simulink model "scara_sim"  (Simulink 8.5)
settings: Solver=ode45  StartTime=0.0  StopTime=1  RelTol=1e-3
values from neighbouring files (symbols this model uses):
  scara = SerialLink(L, 'name', 'scara')    [RunMe_M.m]
libraries: roblocks x3
settings Model: Creator=corkep  LastModifiedBy=ManQi
settings DebuggingCC: SolverPrmCheckMsg=warning  FcnCallInpInsideContextMsg=UseLocalSettings

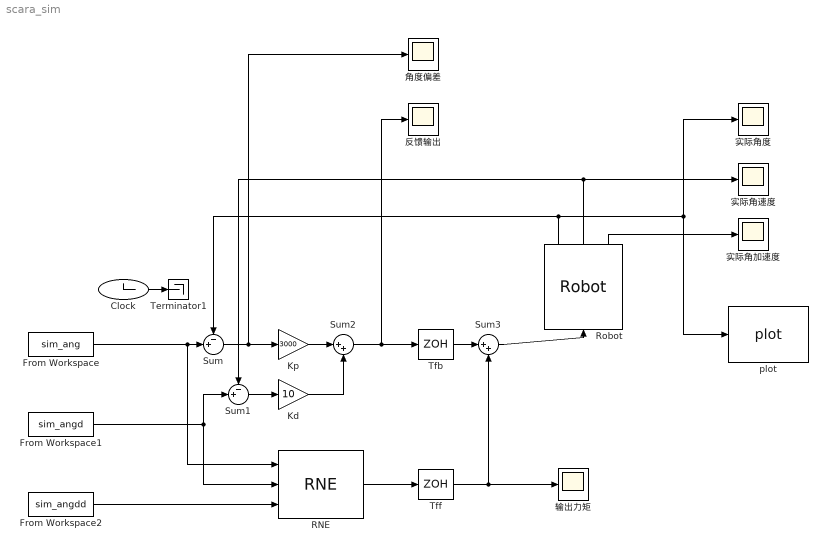
== system scara_sim ==
  Clock : Clock
  From Workspace : FromWorkspace  VariableName=sim_ang  SampleTime=0
  From Workspace1 : FromWorkspace  VariableName=sim_angd  SampleTime=0
  From Workspace2 : FromWorkspace  VariableName=sim_angdd  SampleTime=0
  Kd : Gain  Gain=10  SaturateOnIntegerOverflow=on  OutDataTypeStr=Inherit: Same as input  ParamDataTypeStr=Inherit: Same as input
  Kp : Gain  Gain=3000  SaturateOnIntegerOverflow=on  OutDataTypeStr=Inherit: Same as input  ParamDataTypeStr=Inherit: Same as input
  RNE : roblocks/Dynamics/RNE  robot=scara.nofriction()  grav=[0 0 9.81]
  Robot : roblocks/Dynamics/Robot  robot=scara  q0=start_ang
  Sum : Sum  Inputs=-+|  SaturateOnIntegerOverflow=on  InputSameDT=on  OutDataTypeStr=Inherit: Same as first input
  Sum1 : Sum  Inputs=-+|  SaturateOnIntegerOverflow=on  InputSameDT=on  OutDataTypeStr=Inherit: Same as first input
  Sum2 : Sum  Inputs=|++  SaturateOnIntegerOverflow=on  InputSameDT=on  OutDataTypeStr=Inherit: Same as first input
  Sum3 : Sum  Inputs=|++  SaturateOnIntegerOverflow=on  InputSameDT=on  OutDataTypeStr=Inherit: Same as first input
  Terminator1 : Terminator
  Tfb : ZeroOrderHold  SampleTime=0.005
  Tff : ZeroOrderHold  SampleTime=0.005
  plot : roblocks/Robot Graphics/plot  robot=scara  fps=60  holdplot=on
  反馈输出 : Scope
      settings: YMin=-100  YMax=100  SaveName=ScopeData2
  实际角加速度 : Scope
      settings: YMin=-27.5  YMax=2.5  SaveName=ScopeData4
  实际角度 : Scope
      settings: YMin=-27.5  YMax=2.5  SaveName=ScopeData5
  实际角速度 : Scope
      settings: YMin=-27.5  YMax=2.5  SaveName=ScopeData3
  角度偏差 : Scope
      settings: YMin=-0.04  YMax=0.04
  输出力矩 : Scope
      settings: YMin=-700000  YMax=100000
  wires:
  Kd/1 -> Sum2/2
  Sum/1 -> Kp/1, 角度偏差/1
  Kp/1 -> Sum2/1
  Sum1/1 -> Kd/1
  Sum2/1 -> Tfb/1, 反馈输出/1
  Sum3/1 -> Robot/1
  Robot/1 -> plot/1, 实际角度/1, Sum/1
  Robot/2 -> Sum1/1, 实际角速度/1
  From Workspace/1 -> RNE/1, Sum/2
  From Workspace1/1 -> Sum1/2, RNE/2
  From Workspace2/1 -> RNE/3
  Robot/3 -> 实际角加速度/1
  Tff/1 -> Sum3/2, 输出力矩/1
  Tfb/1 -> Sum3/1
  RNE/1 -> Tff/1
  Clock/1 -> Terminator1/1
